simulink model "hdv_hydroelectropowertrain_model"  (R2026a)
settings: Solver=ode1be  StopTime=simulation_length  FixedStep=tsample  MaxStep=tsample
undefined symbols (not defined in the file): alpha, Apump, available_torque, Bpump, btheta_shaft, C1, consumption, Cpump, dp_lim, E0, E1, E2, E3, E_1, Elog, eta_v_m, eta_v_p, ki_dp_comp, ki_te_comp, kp_ctrl_m, kp_dp_comp, kp_te_comp, Kpump, load_blade_enable, Lpump, M, magnitude, Ncell, Npump, omega_e_rpm_ref, omega_l_max_rpm, q1Kalman, q2Kalman, q3Kalman, Qhr, R0, R1, R_tg, rKalman, rpm_base, rpm_consumption, simulation_length, tau_load, tau_load_max, Tc, torque_base, torque_consumption, torque_friction_base, tsample, v_track1_ref, v_track2_ref, valve_mmorifice_max, xv_m_max
libraries: fl_lib x383, nesl_utility x162, linear_swashplate_ctrl_lib x8, flexshaft_lib x5, bichamber_piston_lib x5, variable_displacement_motor_lib x4, variable_displacement_pump_lib x4, fixed_displacement_pump_lib x4, relief_valve_lib x4, inverse_shuttle_valve_lib x4, hydrostatic_threeway_valve_bichamber_piston_lib x4, hydrostatic_fourway_valve_bichamber_piston_lib x4
(part 4 of 8)

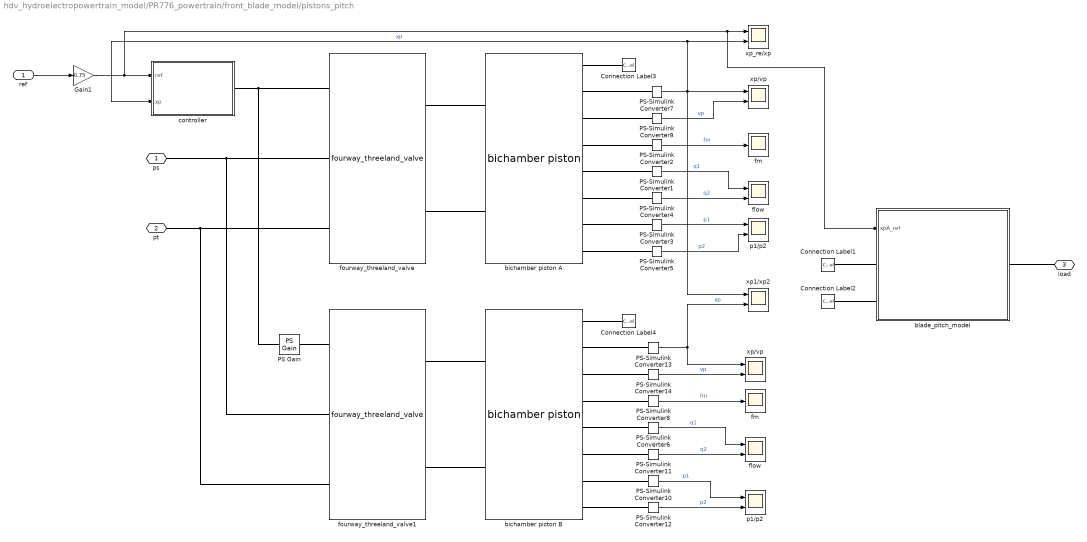
== system hdv_hydroelectropowertrain_model/PR776_powertrain/front_blade_model/pistons_pitch ==
  ref : Inport
  Connection Label1 : ConnectionLabel  Label=A
  Connection Label2 : ConnectionLabel  Label=B
  Connection Label3 : ConnectionLabel  Label=A
  Connection Label4 : ConnectionLabel  Label=B
  Gain1 : Gain  Gain=0.75
  PS Gain : fl_lib/Physical Signals/Functions/PS Gain  gain=-1
  PS-Simulink Converter{1..14} (14 alike) : nesl_utility/PS-Simulink Converter  PhysicalDomain=network_engine_domain  SubClassName=ps_output  LeftPortType=input  RightPortType=output  PseudoPeriodic=off  Frequencies=[]  VectorFormat=1-D array  Unit=inherit  AffineConversion=off
  bichamber piston A : bichamber_piston_lib/bichamber piston  A1=8e-3 m^2  A2=8e-3 m^2  Lp=1.1 m  mp=35 kg  kp=0 N/m  bp=1e3 N/(m/s)  V0=12 l  q1_specify=off  q1_priority=None  q1=0 m^3/s  q1_nominal_specify=off  q1_nominal_value=1  q1_nominal_unit=m^3/s  q2_specify=off  q2_priority=None  q2=0 m^3/s  q2_nominal_specify=off  q2_nominal_value=1  q2_nominal_unit=m^3/s  p1_specify=off  p1_priority=High  p1=0 bar  p1_nominal_specify=off  p1_nominal_value=1  p1_nominal_unit=bar  p2_specify=off  p2_priority=High  p2=0 bar  p2_nominal_specify=off  p2_nominal_value=1  p2_nominal_unit=bar  fp_specify=off  fp_priority=None  fp=0 N  fp_nominal_specify=off  fp_nominal_value=1  fp_nominal_unit=N  vp_specify=off  vp_priority=None  vp=0 m/s  vp_nominal_specify=off  vp_nominal_value=1  vp_nominal_unit=m/s  xp_specify=off  xp_priority=High  xp=0 m  xp_nominal_specify=off  xp_nominal_value=1  xp_nominal_unit=m
  bichamber piston B : bichamber_piston_lib/bichamber piston  A1=8e-3 m^2  A2=8e-3 m^2  Lp=1.1 m  mp=35 kg  kp=0 N/m  bp=1e3 N/(m/s)  V0=12 l  q1_specify=off  q1_priority=None  q1=0 m^3/s  q1_nominal_specify=off  q1_nominal_value=1  q1_nominal_unit=m^3/s  q2_specify=off  q2_priority=None  q2=0 m^3/s  q2_nominal_specify=off  q2_nominal_value=1  q2_nominal_unit=m^3/s  p1_specify=off  p1_priority=High  p1=0 bar  p1_nominal_specify=off  p1_nominal_value=1  p1_nominal_unit=bar  p2_specify=off  p2_priority=High  p2=0 bar  p2_nominal_specify=off  p2_nominal_value=1  p2_nominal_unit=bar  fp_specify=off  fp_priority=None  fp=0 N  fp_nominal_specify=off  fp_nominal_value=1  fp_nominal_unit=N  vp_specify=off  vp_priority=None  vp=0 m/s  vp_nominal_specify=off  vp_nominal_value=1  vp_nominal_unit=m/s  xp_specify=off  xp_priority=High  xp=0 m  xp_nominal_specify=off  xp_nominal_value=1  xp_nominal_unit=m
  blade_pitch_model : Subsystem
  controller : Subsystem
  flow : Scope  NumInputPorts=2
      settings: ActiveDisplayYMinimum=-390.093  ActiveDisplayYMaximum=390.1347
  "flow " : Scope  NumInputPorts=2
      settings: ActiveDisplayYMinimum=-390.093  ActiveDisplayYMaximum=390.1347
  fm : Scope
      settings: ActiveDisplayYMinimum=-672.90251  ActiveDisplayYMaximum=953.14819  DataLoggingVariableName=ScopeData2
  "fm " : Scope
      settings: ActiveDisplayYMinimum=-12251.54126  ActiveDisplayYMaximum=12272.93523  DataLoggingVariableName=ScopeData2
  fourway_threeland_valve : fourway_threeland_valve_lib/fourway_threeland_valve  xv_max=valve_mmorifice_max mm  q1_specify=off  q1_priority=None  q1=0 m^3/s  q1_nominal_specify=off  q1_nominal_unit=m^3/s  q1_nominal_value=1  q2_specify=off  q2_priority=None  q2=0 m^3/s  q2_nominal_specify=off  q2_nominal_unit=m^3/s  q2_nominal_value=1  qin_specify=off  qin_priority=None  qin=0 m^3/s  qin_nominal_specify=off  qin_nominal_unit=m^3/s  qin_nominal_value=1  qout_specify=off  qout_priority=None  qout=0 m^3/s  qout_nominal_specify=off  qout_nominal_unit=m^3/s  qout_nominal_value=1  p1_specify=off  p1_priority=None  p1=0 bar  p1_nominal_specify=off  p1_nominal_unit=bar  p1_nominal_value=1  p2_specify=off  p2_priority=None  p2=0 bar  p2_nominal_specify=off  p2_nominal_unit=bar  p2_nominal_value=1  ps_specify=off  ps_priority=None  ps=0 bar  ps_nominal_specify=off  ps_nominal_unit=bar  ps_nominal_value=1  pt_specify=off  pt_priority=None  pt=0 bar  pt_nominal_specify=off  pt_nominal_unit=bar  pt_nominal_value=1
  fourway_threeland_valve1 : fourway_threeland_valve_lib/fourway_threeland_valve  xv_max=valve_mmorifice_max mm  q1_specify=off  q1_priority=None  q1=0 m^3/s  q1_nominal_specify=off  q1_nominal_unit=m^3/s  q1_nominal_value=1  q2_specify=off  q2_priority=None  q2=0 m^3/s  q2_nominal_specify=off  q2_nominal_unit=m^3/s  q2_nominal_value=1  qin_specify=off  qin_priority=None  qin=0 m^3/s  qin_nominal_specify=off  qin_nominal_unit=m^3/s  qin_nominal_value=1  qout_specify=off  qout_priority=None  qout=0 m^3/s  qout_nominal_specify=off  qout_nominal_unit=m^3/s  qout_nominal_value=1  p1_specify=off  p1_priority=None  p1=0 bar  p1_nominal_specify=off  p1_nominal_unit=bar  p1_nominal_value=1  p2_specify=off  p2_priority=None  p2=0 bar  p2_nominal_specify=off  p2_nominal_unit=bar  p2_nominal_value=1  ps_specify=off  ps_priority=None  ps=0 bar  ps_nominal_specify=off  ps_nominal_unit=bar  ps_nominal_value=1  pt_specify=off  pt_priority=None  pt=0 bar  pt_nominal_specify=off  pt_nominal_unit=bar  pt_nominal_value=1
  p1/p2 : Scope  NumInputPorts=2
      settings: ActiveDisplayYMinimum=-46.741  ActiveDisplayYMaximum=145.78787  DataLoggingVariableName=ScopeData4
  "p1/p2 " : Scope  NumInputPorts=2
      settings: ActiveDisplayYMinimum=-538.19348  ActiveDisplayYMaximum=761.65919  DataLoggingVariableName=ScopeData3
  xp/vp : Scope  NumInputPorts=2
      settings: ActiveDisplayYMinimum=-0.08067  ActiveDisplayYMaximum=1.22604
  "xp/vp " : Scope  NumInputPorts=2
      settings: ActiveDisplayYMinimum=0.8942  ActiveDisplayYMaximum=1.45218  DataLoggingVariableName=ScopeData4
  xp1/xp2 : Scope  NumInputPorts=2
      settings: ActiveDisplayYMinimum=-0.46875  ActiveDisplayYMaximum=0.46875  DataLoggingVariableName=ScopeData6
  xp_re/xp : Scope  NumInputPorts=2
      settings: ActiveDisplayYMinimum=-0.125  ActiveDisplayYMaximum=1.125  DataLoggingVariableName=ScopeData7
  ps : PMIOPort  Side=Left
  pt : PMIOPort  Port=2  Side=Left
  load : PMIOPort  Port=3  Side=Right
  wires:
  PS-Simulink Converter10/1 -> "p1/p2 "/1  "p1"
  PS-Simulink Converter13/1 -> xp1/xp2/2, "xp/vp "/1  "xp"
  PS-Simulink Converter11/1 -> "flow "/2  "q2"
  PS-Simulink Converter14/1 -> "xp/vp "/2  "vp"
  PS-Simulink Converter12/1 -> "p1/p2 "/2  "p2"
  PS-Simulink Converter6/1 -> "flow "/1  "q1"
  PS-Simulink Converter8/1 -> "fm "/1  "fm"
  PS-Simulink Converter2/1 -> fm/1  "fm"
  PS-Simulink Converter1/1 -> flow/1  "q1"
  PS-Simulink Converter5/1 -> p1/p2/2  "p2"
  PS-Simulink Converter9/1 -> xp/vp/2  "vp"
  PS-Simulink Converter4/1 -> flow/2  "q2"
  PS-Simulink Converter7/1 -> xp1/xp2/1, xp/vp/1, controller/2(xp), xp_re/xp/2  "xp"
  PS-Simulink Converter3/1 -> p1/p2/1  "p1"
  ref/1 -> Gain1/1
  Gain1/1 -> controller/1(ref), blade_pitch_model/1(xpA_ref), xp_re/xp/1
  connections:
  bichamber piston B/RConn6 -- PS-Simulink Converter11/LConn1
  bichamber piston B/RConn3 -- PS-Simulink Converter14/LConn1
  bichamber piston B/RConn2 -- PS-Simulink Converter13/LConn1
  bichamber piston B/RConn4 -- PS-Simulink Converter8/LConn1
  bichamber piston B/RConn8 -- PS-Simulink Converter12/LConn1
  bichamber piston B/RConn5 -- PS-Simulink Converter6/LConn1
  bichamber piston B/RConn7 -- PS-Simulink Converter10/LConn1
  fourway_threeland_valve/LConn1 -- PS Gain/LConn1 -- controller/RConn1
  pt/RConn1 -- fourway_threeland_valve/LConn3 -- fourway_threeland_valve1/LConn3
  ps/RConn1 -- fourway_threeland_valve/LConn2 -- fourway_threeland_valve1/LConn2
  bichamber piston A/RConn8 -- PS-Simulink Converter5/LConn1
  bichamber piston A/RConn7 -- PS-Simulink Converter3/LConn1
  bichamber piston A/RConn6 -- PS-Simulink Converter4/LConn1
  bichamber piston A/RConn5 -- PS-Simulink Converter1/LConn1
  bichamber piston A/RConn4 -- PS-Simulink Converter2/LConn1
  bichamber piston A/RConn2 -- PS-Simulink Converter7/LConn1
  bichamber piston A/LConn1 -- fourway_threeland_valve/RConn1
  bichamber piston A/LConn2 -- fourway_threeland_valve/RConn2
  PS Gain/RConn1 -- fourway_threeland_valve1/LConn1
  bichamber piston A/RConn3 -- PS-Simulink Converter9/LConn1
  fourway_threeland_valve1/RConn1 -- bichamber piston B/LConn1
  fourway_threeland_valve1/RConn2 -- bichamber piston B/LConn2
  Connection Label3/LConn1 -- bichamber piston A/RConn1
  bichamber piston B/RConn1 -- Connection Label4/LConn1
  Connection Label1/LConn1 -- blade_pitch_model/LConn1
  Connection Label2/LConn1 -- blade_pitch_model/LConn2
  blade_pitch_model/RConn1 -- load/RConn1

== system hdv_hydroelectropowertrain_model/PR776_powertrain/front_blade_model/pitch_load ==
  Simulink-PS Converter1 : nesl_utility/Simulink-PS Converter  PhysicalDomain=network_engine_domain  SubClassName=ps_input  LeftPortType=input  RightPortType=output  PseudoPeriodic=off  Frequencies=[]  NoiseDistribution=none  NoiseParameters=[]  Unit=N  AffineConversion=on  FilteringAndDerivatives=provide  SimscapeFilterOrder=1  InputFilterTimeConstant=0.001  UdotUserProvided=0
  "pitch_load  " : Subsystem
  load : PMIOPort  Side=Right
  wires:
  "pitch_load  "/1(Out1) -> Simulink-PS Converter1/1  "pitch_load"
  connections:
  load/RConn1 -- Simulink-PS Converter1/RConn1

== system hdv_hydroelectropowertrain_model/PR776_powertrain/front_blade_model/tilt_load ==
  Simulink-PS Converter1 : nesl_utility/Simulink-PS Converter  PhysicalDomain=network_engine_domain  SubClassName=ps_input  LeftPortType=input  RightPortType=output  PseudoPeriodic=off  Frequencies=[]  NoiseDistribution=none  NoiseParameters=[]  Unit=N  AffineConversion=on  FilteringAndDerivatives=provide  SimscapeFilterOrder=1  InputFilterTimeConstant=0.001  UdotUserProvided=0
  "tilt_load  " : Subsystem
  load : PMIOPort  Side=Right
  wires:
  "tilt_load  "/1(Out1) -> Simulink-PS Converter1/1  "tilt_load"
  connections:
  load/RConn1 -- Simulink-PS Converter1/RConn1

== system hdv_hydroelectropowertrain_model/PR776_powertrain/front_blade_model/vertical_load ==
  Blade_load : fl_lib/Mechanical/Mechanical Sources/Ideal Force Source
  Constant : Constant  Value=31878
  Mechanical Translational Reference : fl_lib/Mechanical/Translational Elements/Mechanical Translational Reference
  Simulink-PS Converter1 : nesl_utility/Simulink-PS Converter  PhysicalDomain=network_engine_domain  SubClassName=ps_input  LeftPortType=input  RightPortType=output  PseudoPeriodic=off  Frequencies=[]  NoiseDistribution=none  NoiseParameters=[]  Unit=N  AffineConversion=on  FilteringAndDerivatives=provide  SimscapeFilterOrder=1  InputFilterTimeConstant=0.001  UdotUserProvided=0
  To Workspace6 : ToWorkspace  VariableName=sim_load  SampleTime=Tc
      settings: MaxDataPoints=Nc
  load : Scope
      settings: ActiveDisplayYMinimum=-19625  ActiveDisplayYMaximum=176625  DataLoggingVariableName=ScopeData3
  load_disturbance : Subsystem
  vertical_load : PMIOPort  Side=Left
  wires:
  load_disturbance/1(Out1) -> load/1, To Workspace6/1  "load_force"
  Constant/1 -> Simulink-PS Converter1/1
  connections:
  Mechanical Translational Reference/LConn1 -- Blade_load/RConn2
  Simulink-PS Converter1/RConn1 -- Blade_load/RConn1
  vertical_load/RConn1 -- Blade_load/LConn1

== system hdv_hydroelectropowertrain_model/Vehicle Control System/Engine Anti-Stall/Engine Overload Control ==
  x : Inport
  xref : Inport  Port=2
  1/Ti : Gain  Gain=kp  SaturateOnIntegerOverflow=on  OutDataTypeStr=Inherit: Same as input  ParamDataTypeStr=Inherit: Same as input
  Saturation : Saturate  UpperLimit=sat_pos  LowerLimit=sat_neg
  Sum1 : Sum  Inputs=+++  SaturateOnIntegerOverflow=on
  Sum2 : Sum  Inputs=-+  SaturateOnIntegerOverflow=on
  Sum3 : Sum  Inputs=-+  SaturateOnIntegerOverflow=on
  Unit Delay4 : UnitDelay  SampleTime=tsample
  kp : Gain  Gain=ki*ts  SaturateOnIntegerOverflow=on  OutDataTypeStr=Inherit: Same as input  ParamDataTypeStr=Inherit: Same as input
  u : Outport
  wires:
  Saturation/1 -> Sum3/2, u/1
  Unit Delay4/1 -> Sum1/3
  Sum1/1 -> Saturation/1
  x/1 -> Sum2/1
  Sum3/1 -> Unit Delay4/1
  1/Ti/1 -> Sum3/1, Sum1/1
  Sum2/1 -> 1/Ti/1, kp/1
  kp/1 -> Sum1/2
  xref/1 -> Sum2/2

== system hdv_hydroelectropowertrain_model/Vehicle Control System/Over Pressure Compensation/Pressure Compensation Control A ==
  x : Inport
  xref : Inport  Port=2
  1/Ti : Gain  Gain=kp  SaturateOnIntegerOverflow=on  OutDataTypeStr=Inherit: Same as input  ParamDataTypeStr=Inherit: Same as input
  Saturation : Saturate  UpperLimit=sat_pos  LowerLimit=sat_neg
  Sum1 : Sum  Inputs=+++  SaturateOnIntegerOverflow=on
  Sum2 : Sum  Inputs=-+  SaturateOnIntegerOverflow=on
  Sum3 : Sum  Inputs=-+  SaturateOnIntegerOverflow=on
  Unit Delay4 : UnitDelay  SampleTime=tsample
  kp : Gain  Gain=ki*ts  SaturateOnIntegerOverflow=on  OutDataTypeStr=Inherit: Same as input  ParamDataTypeStr=Inherit: Same as input
  u : Outport
  wires:
  xref/1 -> Sum2/2
  kp/1 -> Sum1/2
  1/Ti/1 -> Sum1/1, Sum3/1
  Sum3/1 -> Unit Delay4/1
  x/1 -> Sum2/1
  Sum1/1 -> Saturation/1
  Unit Delay4/1 -> Sum1/3
  Saturation/1 -> u/1, Sum3/2
  Sum2/1 -> 1/Ti/1, kp/1

== system hdv_hydroelectropowertrain_model/Vehicle Control System/Over Pressure Compensation/Pressure Compensation Control B ==
  x : Inport
  xref : Inport  Port=2
  1/Ti : Gain  Gain=kp  SaturateOnIntegerOverflow=on  OutDataTypeStr=Inherit: Same as input  ParamDataTypeStr=Inherit: Same as input
  Saturation : Saturate  UpperLimit=sat_pos  LowerLimit=sat_neg
  Sum1 : Sum  Inputs=+++  SaturateOnIntegerOverflow=on
  Sum2 : Sum  Inputs=-+  SaturateOnIntegerOverflow=on
  Sum3 : Sum  Inputs=-+  SaturateOnIntegerOverflow=on
  Unit Delay4 : UnitDelay  SampleTime=tsample
  kp : Gain  Gain=ki*ts  SaturateOnIntegerOverflow=on  OutDataTypeStr=Inherit: Same as input  ParamDataTypeStr=Inherit: Same as input
  u : Outport
  wires:
  Saturation/1 -> Sum3/2, u/1
  Unit Delay4/1 -> Sum1/3
  Sum1/1 -> Saturation/1
  x/1 -> Sum2/1
  Sum3/1 -> Unit Delay4/1
  1/Ti/1 -> Sum3/1, Sum1/1
  Sum2/1 -> 1/Ti/1, kp/1
  kp/1 -> Sum1/2
  xref/1 -> Sum2/2

== system hdv_hydroelectropowertrain_model/Vehicle Control System/Over Pressure Compensation/direction1 ==
  In1 : Inport
  Product : Product
  Out1 : Outport
  wires:
  In1/1 -> Product/1
  Product/1 -> Out1/1
  [direction_RT] -> Product/2

== system hdv_hydroelectropowertrain_model/Vehicle Control System/Over Pressure Compensation/direction2 ==
  In1 : Inport
  Product : Product
  Out1 : Outport
  wires:
  Product/1 -> Out1/1
  In1/1 -> Product/1
  [direction_LT] -> Product/2

== system hdv_hydroelectropowertrain_model/Vehicle Control System/lineA_compensations/direction_RT ==
  In1 : Inport
  Product : Product
  ETComp : Outport
  wires:
  Product/1 -> ETComp/1
  In1/1 -> Product/1
  [direction_RT] -> Product/2

== system hdv_hydroelectropowertrain_model/Vehicle Control System/lineB_compensations /direction_LT ==
  In1 : Inport
  Product : Product
  ETComp : Outport
  wires:
  Product/1 -> ETComp/1
  In1/1 -> Product/1
  [direction_LT] -> Product/2

== system hdv_hydroelectropowertrain_model/Vehicle Control System/synch_overspeed_management/Maximum Speed Control ==
  x : Inport
  xref : Inport  Port=2
  1/Ti : Gain  Gain=kp  SaturateOnIntegerOverflow=on  OutDataTypeStr=Inherit: Same as input  ParamDataTypeStr=Inherit: Same as input
  Saturation : Saturate  UpperLimit=sat_pos  LowerLimit=sat_neg
  Sum1 : Sum  Inputs=+++  SaturateOnIntegerOverflow=on
  Sum2 : Sum  Inputs=-+  SaturateOnIntegerOverflow=on
  Sum3 : Sum  Inputs=-+  SaturateOnIntegerOverflow=on
  Unit Delay4 : UnitDelay  SampleTime=ts
  direction_lineA : Subsystem
  kp : Gain  Gain=ki*tsample  SaturateOnIntegerOverflow=on  OutDataTypeStr=Inherit: Same as input  ParamDataTypeStr=Inherit: Same as input
  u : Outport
  wires:
  xref/1 -> Sum2/2
  kp/1 -> Sum1/2
  1/Ti/1 -> Sum1/1, Sum3/1
  Sum3/1 -> Unit Delay4/1
  x/1 -> Sum2/1
  Sum1/1 -> Saturation/1
  Unit Delay4/1 -> Sum1/3
  Saturation/1 -> direction_lineA/1(In1), Sum3/2
  Sum2/1 -> kp/1, 1/Ti/1
  direction_lineA/1(u) -> u/1

== system hdv_hydroelectropowertrain_model/Vehicle Control System/synch_overspeed_management/Steering Reference Control ==
  x : Inport
  xref : Inport  Port=2
  1/Ti : Gain  Gain=kp  SaturateOnIntegerOverflow=on  OutDataTypeStr=Inherit: Same as input  ParamDataTypeStr=Inherit: Same as input
  Saturation : Saturate  UpperLimit=sat_pos  LowerLimit=sat_neg
  Sum1 : Sum  Inputs=+++  SaturateOnIntegerOverflow=on
  Sum2 : Sum  Inputs=-+  SaturateOnIntegerOverflow=on
  Sum3 : Sum  Inputs=-+  SaturateOnIntegerOverflow=on
  Unit Delay4 : UnitDelay  SampleTime=tsample
  kp : Gain  Gain=ki*ts  SaturateOnIntegerOverflow=on  OutDataTypeStr=Inherit: Same as input  ParamDataTypeStr=Inherit: Same as input
  u : Outport
  wires:
  Saturation/1 -> Sum3/2, u/1
  Unit Delay4/1 -> Sum1/3
  Sum1/1 -> Saturation/1
  x/1 -> Sum2/1
  Sum3/1 -> Unit Delay4/1
  1/Ti/1 -> Sum3/1, Sum1/1
  Sum2/1 -> 1/Ti/1, kp/1
  kp/1 -> Sum1/2
  xref/1 -> Sum2/2

== system hdv_hydroelectropowertrain_model/PR776_powertrain/Hydrostatic_powertrain/driveine_LD1/pressure_charge_system_LD ==
  Hydraulic Flow Rate Sensor : fl_lib/Hydraulic/Hydraulic Sensors/Hydraulic Flow Rate Sensor
  Hydraulic Flow Rate Sensor1 : fl_lib/Hydraulic/Hydraulic Sensors/Hydraulic Flow Rate Sensor
  Hydraulic Pressure Sensor{1..4} (4 alike) : fl_lib/Hydraulic/Hydraulic Sensors/Hydraulic Pressure Sensor
  Hydraulic Reference1 : fl_lib/Hydraulic/Hydraulic Elements/Hydraulic Reference
  Hydraulic Reference2 : fl_lib/Hydraulic/Hydraulic Elements/Hydraulic Reference
  Hydraulic Reference3 : fl_lib/Hydraulic/Hydraulic Elements/Hydraulic Reference
  Mux : Mux  Inputs=2
  PS-Simulink Converter : nesl_utility/PS-Simulink Converter  PhysicalDomain=network_engine_domain  SubClassName=ps_output  LeftPortType=input  RightPortType=output  PseudoPeriodic=off  Frequencies=[]  VectorFormat=1-D array  Unit=l/min  AffineConversion=on
  PS-Simulink Converter{1..3,5} (4 alike) : nesl_utility/PS-Simulink Converter  PhysicalDomain=network_engine_domain  SubClassName=ps_output  LeftPortType=input  RightPortType=output  PseudoPeriodic=off  Frequencies=[]  VectorFormat=1-D array  Unit=bar  AffineConversion=on
  PS-Simulink Converter4 : nesl_utility/PS-Simulink Converter  PhysicalDomain=network_engine_domain  SubClassName=ps_output  LeftPortType=input  RightPortType=output  PseudoPeriodic=off  Frequencies=[]  VectorFormat=1-D array  Unit=l/min  AffineConversion=on
  Scope1 : Scope  NumInputPorts=2
      settings: SampleTime=tsample  ActiveDisplayYMinimum=-171.1725  ActiveDisplayYMaximum=527.07344  DataLoggingVariableName=ScopeData2
  Scope2 : Scope  NumInputPorts=2
      settings: SampleTime=tsample  ActiveDisplayYMinimum=-2.39042  ActiveDisplayYMaximum=21.51378  DataLoggingVariableName=ScopeData2
  Scope3 : Scope  NumInputPorts=2
      settings: SampleTime=tsample  ActiveDisplayYMinimum=-2.35304  ActiveDisplayYMaximum=21.17734
  Subsystem : Subsystem
  hydro_check_valve1 : Subsystem
      settings: PortSchema="{\"entries\":[{\"content\":{\"sides\":[{\"content\":{\"connectorIds\":[]},\"type\":\"ConnectorPlacement.EquallySpacedRectSide\",\"uuid\":\"a69fbb91-2279-4dfd-af6f-16497d5f1538\"},{\"content\":{\"connectorIds\":[],\"side\":\"RIGHT\"},\"type\":\"ConnectorPlacement.EquallySpacedRectSide\",\"uuid\":\"52e95d44-b7af-4ccc-8556-a2abd2e724e0\"},{\"content\":{\"connectorIds\":[\"LConn1\"],\"side\":\"TOP\"},\"type\":\"ConnectorPlacement.EquallySpacedRectSide\",\"uuid\":\"2d8c071e-4cd0-4b83-8d45-c175cb858754\"},{\"content\":{\"connectorIds\":[\"RConn1\"],\"side\":\"BOTTOM\"},\"type\":\"ConnectorPlacement.EquallySpacedRectSide\",\"uuid\":\"1baec9dc-757c-4f21-904a-6fc08de72ce1\"}]},\"type\":\"ConnectorPlacement.EquallySpacedConnector\",\"uuid\":\"76990e53-6cb0-4bfe-8c9e-427c41b785f2\"}],\"packageUris\":[\"http://schema.mathworks.com/mf0/Connector/19700101\"],\"version\":\"1.0\"}"
  hydro_check_valve2 : Subsystem
      settings: PortSchema="{\"entries\":[{\"content\":{\"sides\":[{\"content\":{\"connectorIds\":[]},\"type\":\"ConnectorPlacement.EquallySpacedRectSide\",\"uuid\":\"a69fbb91-2279-4dfd-af6f-16497d5f1538\"},{\"content\":{\"connectorIds\":[],\"side\":\"RIGHT\"},\"type\":\"ConnectorPlacement.EquallySpacedRectSide\",\"uuid\":\"52e95d44-b7af-4ccc-8556-a2abd2e724e0\"},{\"content\":{\"connectorIds\":[\"LConn1\"],\"side\":\"TOP\"},\"type\":\"ConnectorPlacement.EquallySpacedRectSide\",\"uuid\":\"2d8c071e-4cd0-4b83-8d45-c175cb858754\"},{\"content\":{\"connectorIds\":[\"RConn1\"],\"side\":\"BOTTOM\"},\"type\":\"ConnectorPlacement.EquallySpacedRectSide\",\"uuid\":\"1baec9dc-757c-4f21-904a-6fc08de72ce1\"}]},\"type\":\"ConnectorPlacement.EquallySpacedConnector\",\"uuid\":\"76990e53-6cb0-4bfe-8c9e-427c41b785f2\"}],\"packageUris\":[\"http://schema.mathworks.com/mf0/Connector/19700101\"],\"version\":\"1.0\"}"
  inverse shuttle valve : inverse_shuttle_valve_lib/inverse shuttle valve  pnom=32 bar  dp_crack=0 bar  dp_reg=0 bar  x_rv_max=2 mm  a0=(2*pi*10)^2 1/s^2  a1=2*2*pi*10 1/s  leak=5e-12 m^3/s/Pa  qA_specify=off  qA_priority=None  qA=0 m^3/s  qA_nominal_specify=off  qA_nominal_unit=m^3/s  qA_nominal_value=1  qB_specify=off  qB_priority=None  qB=0 m^3/s  qB_nominal_specify=off  qB_nominal_unit=m^3/s  qB_nominal_value=1  qP_specify=off  qP_priority=None  qP=0 m^3/s  qP_nominal_specify=off  qP_nominal_unit=m^3/s  qP_nominal_value=1  dp_specify=off  dp_priority=None  dp=0 Pa  dp_nominal_specify=off  dp_nominal_unit=Pa  dp_nominal_value=1  dpAP_specify=off  dpAP_priority=None  dpAP=0 Pa  dpAP_nominal_specify=off  dpAP_nominal_unit=Pa  dpAP_nominal_value=1  dpBP_specify=off  dpBP_priority=None  dpBP=0 Pa  dpBP_nominal_specify=off  dpBP_nominal_unit=Pa  dpBP_nominal_value=1  x_rv_AP_specify=off  x_rv_AP_priority=None  x_rv_AP=0 m  x_rv_AP_nominal_specify=off  x_rv_AP_nominal_unit=m  x_rv_AP_nominal_value=1  x_rv_BP_specify=off  x_rv_BP_priority=None  x_rv_BP=0 m  x_rv_BP_nominal_specify=off  x_rv_BP_nominal_unit=m  x_rv_BP_nominal_value=1  x_rv_AP_flt_specify=off  x_rv_AP_flt_priority=None  x_rv_AP_flt=0 m  x_rv_AP_flt_nominal_specify=off  x_rv_AP_flt_nominal_unit=m  x_rv_AP_flt_nominal_value=1  x_rv_BP_flt_specify=off  x_rv_BP_flt_priority=None  x_rv_BP_flt=0 m  x_rv_BP_flt_nominal_specify=off  x_rv_BP_flt_nominal_unit=m  x_rv_BP_flt_nominal_value=1
  A : PMIOPort  Side=Left
  B : PMIOPort  Port=2  Side=Right
  D : PMIOPort  Port=3  Side=Right
  wires:
  PS-Simulink Converter5/1 -> Scope3/2  "dp"
  PS-Simulink Converter4/1 -> Scope3/1  "qT_ishuttle"
  PS-Simulink Converter3/1 -> Scope2/2  "pCharge"
  PS-Simulink Converter/1 -> Scope1/2, Scope2/1  "qcharge"
  Mux/1 -> Scope1/1
  PS-Simulink Converter1/1 -> Mux/1  "pB"
  PS-Simulink Converter2/1 -> Mux/2  "pA"
  connections:
  PS-Simulink Converter5/LConn1 -- Hydraulic Pressure Sensor4/RConn2
  Hydraulic Flow Rate Sensor1/RConn1 -- PS-Simulink Converter4/LConn1
  Hydraulic Flow Rate Sensor1/RConn2 -- Hydraulic Reference3/LConn1
  Hydraulic Reference2/LConn1 -- Hydraulic Pressure Sensor3/RConn1
  Hydraulic Pressure Sensor3/RConn2 -- PS-Simulink Converter3/LConn1
  Subsystem/LConn1 -- D/RConn1
  Hydraulic Flow Rate Sensor/LConn1 -- Subsystem/RConn1 -- Hydraulic Pressure Sensor3/LConn1
  Hydraulic Flow Rate Sensor/RConn1 -- PS-Simulink Converter/LConn1
  Hydraulic Pressure Sensor2/RConn2 -- PS-Simulink Converter2/LConn1
  Hydraulic Pressure Sensor1/RConn2 -- PS-Simulink Converter1/LConn1
  Hydraulic Pressure Sensor1/RConn1 -- Hydraulic Reference1/LConn1 -- Hydraulic Pressure Sensor2/RConn1
  Hydraulic Pressure Sensor4/RConn1 -- Hydraulic Pressure Sensor1/LConn1 -- B/RConn1 -- inverse shuttle valve/LConn2 -- hydro_check_valve2/RConn1
  Hydraulic Pressure Sensor4/LConn1 -- Hydraulic Pressure Sensor2/LConn1 -- A/RConn1 -- inverse shuttle valve/LConn1 -- hydro_check_valve1/RConn1
  hydro_check_valve1/LConn1 -- Hydraulic Flow Rate Sensor/RConn2 -- hydro_check_valve2/LConn1
  inverse shuttle valve/RConn1 -- Hydraulic Flow Rate Sensor1/LConn1

== system hdv_hydroelectropowertrain_model/PR776_powertrain/Hydrostatic_powertrain/driveine_LD1/vd_ctrl_motor_LD ==
  vd_ref : Inport
  Linear swashplate ctrl2 : linear_swashplate_ctrl_lib/Linear swashplate ctrl  Commented=on  a12=1 1/s  b2=1 1/m/s  k1=100 m  k2=20.5 m  N=5 m  kv=20  xv_specify=off  xv_priority=None  xv=0 m  xv_nominal_specify=off  xv_nominal_unit=m  xv_nominal_value=1  D1_specify=off  D1_priority=None  D1=0  D1_nominal_specify=off  D1_nominal_unit=1  D1_nominal_value=1  D2_specify=off  D2_priority=None  D2=0  D2_nominal_specify=off  D2_nominal_unit=1  D2_nominal_value=1
  PS-Simulink Converter : nesl_utility/PS-Simulink Converter  PhysicalDomain=network_engine_domain  SubClassName=ps_output  LeftPortType=input  RightPortType=output  PseudoPeriodic=off  Frequencies=[]  VectorFormat=1-D array  Unit=inherit  AffineConversion=off
  Scope : Scope  NumInputPorts=2
      settings: ActiveDisplayYMinimum=0.29414  ActiveDisplayYMaximum=1.07846  DataLoggingVariableName=ScopeData3
  Simulink-PS Converter3 : nesl_utility/Simulink-PS Converter  Commented=on  PhysicalDomain=network_engine_domain  SubClassName=ps_input  LeftPortType=input  RightPortType=output  PseudoPeriodic=off  Frequencies=[]  NoiseDistribution=none  NoiseParameters=[]  Unit=1  AffineConversion=off  FilteringAndDerivatives=provide  SimscapeFilterOrder=1  InputFilterTimeConstant=0.001  UdotUserProvided=0
  hose3 : Subsystem
  servo motor LD : Subsystem
  vd : PMIOPort  Side=Right
  pS : PMIOPort  Port=2  Side=Left
  pT : PMIOPort  Port=3  Side=Left
  wires:
  PS-Simulink Converter/1 -> Scope/2
  vd_ref/1 -> servo motor LD/1(displacement reference pu), Scope/1, Simulink-PS Converter3/1
  connections:
  Simulink-PS Converter3/RConn1 -- Linear swashplate ctrl2/LConn1
  pS/RConn1 -- hose3/LConn1
  pT/RConn1 -- hose3/LConn2
  hose3/RConn1 -- servo motor LD/LConn1
  hose3/RConn2 -- servo motor LD/LConn2
  servo motor LD/RConn1 -- PS-Simulink Converter/LConn1 -- vd/RConn1

== system hdv_hydroelectropowertrain_model/PR776_powertrain/Hydrostatic_powertrain/driveine_LD1/vd_ctrl_pump_LD ==
  vd_ref : Inport
  Linear swashplate ctrl2 : linear_swashplate_ctrl_lib/Linear swashplate ctrl  Commented=on  a12=1 1/s  b2=1 1/m/s  k1=100 m  k2=20.5 m  N=5 m  kv=20  xv_specify=off  xv_priority=None  xv=0 m  xv_nominal_specify=off  xv_nominal_unit=m  xv_nominal_value=1  D1_specify=off  D1_priority=None  D1=0  D1_nominal_specify=off  D1_nominal_unit=1  D1_nominal_value=1  D2_specify=off  D2_priority=None  D2=0  D2_nominal_specify=off  D2_nominal_unit=1  D2_nominal_value=1
  Simulink-PS Converter3 : nesl_utility/Simulink-PS Converter  Commented=on  PhysicalDomain=network_engine_domain  SubClassName=ps_input  LeftPortType=input  RightPortType=output  PseudoPeriodic=off  Frequencies=[]  NoiseDistribution=none  NoiseParameters=[]  Unit=1  AffineConversion=off  FilteringAndDerivatives=provide  SimscapeFilterOrder=1  InputFilterTimeConstant=0.001  UdotUserProvided=0
  hose3 : Subsystem
  servo pump RD : Subsystem
  vd : PMIOPort  Side=Right
  pS : PMIOPort  Port=2  Side=Left
  pT : PMIOPort  Port=3  Side=Left
  wires:
  vd_ref/1 -> Simulink-PS Converter3/1, servo pump RD/1(displacement reference pu)
  connections:
  pT/RConn1 -- hose3/LConn2
  pS/RConn1 -- hose3/LConn1
  servo pump RD/LConn1 -- hose3/RConn1
  servo pump RD/LConn2 -- hose3/RConn2
  Simulink-PS Converter3/RConn1 -- Linear swashplate ctrl2/LConn1
  servo pump RD/RConn1 -- vd/RConn1

== system hdv_hydroelectropowertrain_model/PR776_powertrain/Hydrostatic_powertrain/driveine_LD2/pressure_charge_system_LD ==
  Hydraulic Flow Rate Sensor : fl_lib/Hydraulic/Hydraulic Sensors/Hydraulic Flow Rate Sensor
  Hydraulic Flow Rate Sensor1 : fl_lib/Hydraulic/Hydraulic Sensors/Hydraulic Flow Rate Sensor
  Hydraulic Pressure Sensor{1..4} (4 alike) : fl_lib/Hydraulic/Hydraulic Sensors/Hydraulic Pressure Sensor
  Hydraulic Reference1 : fl_lib/Hydraulic/Hydraulic Elements/Hydraulic Reference
  Hydraulic Reference2 : fl_lib/Hydraulic/Hydraulic Elements/Hydraulic Reference
  Hydraulic Reference3 : fl_lib/Hydraulic/Hydraulic Elements/Hydraulic Reference
  Mux : Mux  Inputs=2
  PS-Simulink Converter : nesl_utility/PS-Simulink Converter  PhysicalDomain=network_engine_domain  SubClassName=ps_output  LeftPortType=input  RightPortType=output  PseudoPeriodic=off  Frequencies=[]  VectorFormat=1-D array  Unit=l/min  AffineConversion=on
  PS-Simulink Converter{1..3,5} (4 alike) : nesl_utility/PS-Simulink Converter  PhysicalDomain=network_engine_domain  SubClassName=ps_output  LeftPortType=input  RightPortType=output  PseudoPeriodic=off  Frequencies=[]  VectorFormat=1-D array  Unit=bar  AffineConversion=on
  PS-Simulink Converter4 : nesl_utility/PS-Simulink Converter  PhysicalDomain=network_engine_domain  SubClassName=ps_output  LeftPortType=input  RightPortType=output  PseudoPeriodic=off  Frequencies=[]  VectorFormat=1-D array  Unit=l/min  AffineConversion=on
  Scope1 : Scope  NumInputPorts=2
      settings: SampleTime=tsample  ActiveDisplayYMinimum=-171.1725  ActiveDisplayYMaximum=527.07344  DataLoggingVariableName=ScopeData2
  Scope2 : Scope  NumInputPorts=2
      settings: SampleTime=tsample  ActiveDisplayYMinimum=-2.39042  ActiveDisplayYMaximum=21.51378  DataLoggingVariableName=ScopeData2
  Scope3 : Scope  NumInputPorts=2
      settings: SampleTime=tsample  ActiveDisplayYMinimum=-2.35304  ActiveDisplayYMaximum=21.17734
  Subsystem : Subsystem
  hydro_check_valve1 : Subsystem
      settings: PortSchema="{\"entries\":[{\"content\":{\"sides\":[{\"content\":{\"connectorIds\":[]},\"type\":\"ConnectorPlacement.EquallySpacedRectSide\",\"uuid\":\"a69fbb91-2279-4dfd-af6f-16497d5f1538\"},{\"content\":{\"connectorIds\":[],\"side\":\"RIGHT\"},\"type\":\"ConnectorPlacement.EquallySpacedRectSide\",\"uuid\":\"52e95d44-b7af-4ccc-8556-a2abd2e724e0\"},{\"content\":{\"connectorIds\":[\"LConn1\"],\"side\":\"TOP\"},\"type\":\"ConnectorPlacement.EquallySpacedRectSide\",\"uuid\":\"2d8c071e-4cd0-4b83-8d45-c175cb858754\"},{\"content\":{\"connectorIds\":[\"RConn1\"],\"side\":\"BOTTOM\"},\"type\":\"ConnectorPlacement.EquallySpacedRectSide\",\"uuid\":\"1baec9dc-757c-4f21-904a-6fc08de72ce1\"}]},\"type\":\"ConnectorPlacement.EquallySpacedConnector\",\"uuid\":\"76990e53-6cb0-4bfe-8c9e-427c41b785f2\"}],\"packageUris\":[\"http://schema.mathworks.com/mf0/Connector/19700101\"],\"version\":\"1.0\"}"
  hydro_check_valve2 : Subsystem
      settings: PortSchema="{\"entries\":[{\"content\":{\"sides\":[{\"content\":{\"connectorIds\":[]},\"type\":\"ConnectorPlacement.EquallySpacedRectSide\",\"uuid\":\"a69fbb91-2279-4dfd-af6f-16497d5f1538\"},{\"content\":{\"connectorIds\":[],\"side\":\"RIGHT\"},\"type\":\"ConnectorPlacement.EquallySpacedRectSide\",\"uuid\":\"52e95d44-b7af-4ccc-8556-a2abd2e724e0\"},{\"content\":{\"connectorIds\":[\"LConn1\"],\"side\":\"TOP\"},\"type\":\"ConnectorPlacement.EquallySpacedRectSide\",\"uuid\":\"2d8c071e-4cd0-4b83-8d45-c175cb858754\"},{\"content\":{\"connectorIds\":[\"RConn1\"],\"side\":\"BOTTOM\"},\"type\":\"ConnectorPlacement.EquallySpacedRectSide\",\"uuid\":\"1baec9dc-757c-4f21-904a-6fc08de72ce1\"}]},\"type\":\"ConnectorPlacement.EquallySpacedConnector\",\"uuid\":\"76990e53-6cb0-4bfe-8c9e-427c41b785f2\"}],\"packageUris\":[\"http://schema.mathworks.com/mf0/Connector/19700101\"],\"version\":\"1.0\"}"
  inverse shuttle valve : inverse_shuttle_valve_lib/inverse shuttle valve  pnom=32 bar  dp_crack=0 bar  dp_reg=0 bar  x_rv_max=2 mm  a0=(2*pi*10)^2 1/s^2  a1=2*2*pi*10 1/s  leak=5e-12 m^3/s/Pa  qA_specify=off  qA_priority=None  qA=0 m^3/s  qA_nominal_specify=off  qA_nominal_unit=m^3/s  qA_nominal_value=1  qB_specify=off  qB_priority=None  qB=0 m^3/s  qB_nominal_specify=off  qB_nominal_unit=m^3/s  qB_nominal_value=1  qP_specify=off  qP_priority=None  qP=0 m^3/s  qP_nominal_specify=off  qP_nominal_unit=m^3/s  qP_nominal_value=1  dp_specify=off  dp_priority=None  dp=0 Pa  dp_nominal_specify=off  dp_nominal_unit=Pa  dp_nominal_value=1  dpAP_specify=off  dpAP_priority=None  dpAP=0 Pa  dpAP_nominal_specify=off  dpAP_nominal_unit=Pa  dpAP_nominal_value=1  dpBP_specify=off  dpBP_priority=None  dpBP=0 Pa  dpBP_nominal_specify=off  dpBP_nominal_unit=Pa  dpBP_nominal_value=1  x_rv_AP_specify=off  x_rv_AP_priority=None  x_rv_AP=0 m  x_rv_AP_nominal_specify=off  x_rv_AP_nominal_unit=m  x_rv_AP_nominal_value=1  x_rv_BP_specify=off  x_rv_BP_priority=None  x_rv_BP=0 m  x_rv_BP_nominal_specify=off  x_rv_BP_nominal_unit=m  x_rv_BP_nominal_value=1  x_rv_AP_flt_specify=off  x_rv_AP_flt_priority=None  x_rv_AP_flt=0 m  x_rv_AP_flt_nominal_specify=off  x_rv_AP_flt_nominal_unit=m  x_rv_AP_flt_nominal_value=1  x_rv_BP_flt_specify=off  x_rv_BP_flt_priority=None  x_rv_BP_flt=0 m  x_rv_BP_flt_nominal_specify=off  x_rv_BP_flt_nominal_unit=m  x_rv_BP_flt_nominal_value=1
  A : PMIOPort  Side=Left
  B : PMIOPort  Port=2  Side=Right
  D : PMIOPort  Port=3  Side=Right
  wires:
  PS-Simulink Converter2/1 -> Mux/2  "pA"
  PS-Simulink Converter1/1 -> Mux/1  "pB"
  Mux/1 -> Scope1/1
  PS-Simulink Converter/1 -> Scope2/1, Scope1/2  "qcharge"
  PS-Simulink Converter3/1 -> Scope2/2  "pCharge"
  PS-Simulink Converter4/1 -> Scope3/1  "qT_ishuttle"
  PS-Simulink Converter5/1 -> Scope3/2  "dp"
  connections:
  inverse shuttle valve/RConn1 -- Hydraulic Flow Rate Sensor1/LConn1
  hydro_check_valve2/LConn1 -- Hydraulic Flow Rate Sensor/RConn2 -- hydro_check_valve1/LConn1
  hydro_check_valve1/RConn1 -- inverse shuttle valve/LConn1 -- A/RConn1 -- Hydraulic Pressure Sensor2/LConn1 -- Hydraulic Pressure Sensor4/LConn1
  hydro_check_valve2/RConn1 -- inverse shuttle valve/LConn2 -- B/RConn1 -- Hydraulic Pressure Sensor1/LConn1 -- Hydraulic Pressure Sensor4/RConn1
  Hydraulic Pressure Sensor2/RConn1 -- Hydraulic Reference1/LConn1 -- Hydraulic Pressure Sensor1/RConn1
  Hydraulic Pressure Sensor1/RConn2 -- PS-Simulink Converter1/LConn1
  Hydraulic Pressure Sensor2/RConn2 -- PS-Simulink Converter2/LConn1
  Hydraulic Flow Rate Sensor/RConn1 -- PS-Simulink Converter/LConn1
  Hydraulic Pressure Sensor3/LConn1 -- Subsystem/RConn1 -- Hydraulic Flow Rate Sensor/LConn1
  Subsystem/LConn1 -- D/RConn1
  Hydraulic Pressure Sensor3/RConn2 -- PS-Simulink Converter3/LConn1
  Hydraulic Reference2/LConn1 -- Hydraulic Pressure Sensor3/RConn1
  Hydraulic Flow Rate Sensor1/RConn2 -- Hydraulic Reference3/LConn1
  Hydraulic Flow Rate Sensor1/RConn1 -- PS-Simulink Converter4/LConn1
  PS-Simulink Converter5/LConn1 -- Hydraulic Pressure Sensor4/RConn2

== system hdv_hydroelectropowertrain_model/PR776_powertrain/Hydrostatic_powertrain/driveine_LD2/vd_ctrl_motor_LD ==
  vd_ref : Inport
  Linear swashplate ctrl2 : linear_swashplate_ctrl_lib/Linear swashplate ctrl  Commented=on  a12=1 1/s  b2=1 1/m/s  k1=100 m  k2=20.5 m  N=5 m  kv=20  xv_specify=off  xv_priority=None  xv=0 m  xv_nominal_specify=off  xv_nominal_unit=m  xv_nominal_value=1  D1_specify=off  D1_priority=None  D1=0  D1_nominal_specify=off  D1_nominal_unit=1  D1_nominal_value=1  D2_specify=off  D2_priority=None  D2=0  D2_nominal_specify=off  D2_nominal_unit=1  D2_nominal_value=1
  PS-Simulink Converter : nesl_utility/PS-Simulink Converter  PhysicalDomain=network_engine_domain  SubClassName=ps_output  LeftPortType=input  RightPortType=output  PseudoPeriodic=off  Frequencies=[]  VectorFormat=1-D array  Unit=inherit  AffineConversion=off
  Scope : Scope  NumInputPorts=2
      settings: ActiveDisplayYMinimum=0.29414  ActiveDisplayYMaximum=1.07846  DataLoggingVariableName=ScopeData3
  Simulink-PS Converter3 : nesl_utility/Simulink-PS Converter  Commented=on  PhysicalDomain=network_engine_domain  SubClassName=ps_input  LeftPortType=input  RightPortType=output  PseudoPeriodic=off  Frequencies=[]  NoiseDistribution=none  NoiseParameters=[]  Unit=1  AffineConversion=off  FilteringAndDerivatives=provide  SimscapeFilterOrder=1  InputFilterTimeConstant=0.001  UdotUserProvided=0
  hose3 : Subsystem
  servo motor LD : Subsystem
  vd : PMIOPort  Side=Right
  pS : PMIOPort  Port=2  Side=Left
  pT : PMIOPort  Port=3  Side=Left
  wires:
  vd_ref/1 -> Simulink-PS Converter3/1, Scope/1, servo motor LD/1(displacement reference pu)
  PS-Simulink Converter/1 -> Scope/2
  connections:
  vd/RConn1 -- PS-Simulink Converter/LConn1 -- servo motor LD/RConn1
  hose3/RConn2 -- servo motor LD/LConn2
  hose3/RConn1 -- servo motor LD/LConn1
  pT/RConn1 -- hose3/LConn2
  pS/RConn1 -- hose3/LConn1
  Simulink-PS Converter3/RConn1 -- Linear swashplate ctrl2/LConn1

== system hdv_hydroelectropowertrain_model/PR776_powertrain/Hydrostatic_powertrain/driveine_LD2/vd_ctrl_pump_LD ==
  vd_ref : Inport
  Linear swashplate ctrl2 : linear_swashplate_ctrl_lib/Linear swashplate ctrl  Commented=on  a12=1 1/s  b2=1 1/m/s  k1=100 m  k2=20.5 m  N=5 m  kv=20  xv_specify=off  xv_priority=None  xv=0 m  xv_nominal_specify=off  xv_nominal_unit=m  xv_nominal_value=1  D1_specify=off  D1_priority=None  D1=0  D1_nominal_specify=off  D1_nominal_unit=1  D1_nominal_value=1  D2_specify=off  D2_priority=None  D2=0  D2_nominal_specify=off  D2_nominal_unit=1  D2_nominal_value=1
      settings: InternalSimscapePortConfiguration="{\"Bottom\":[],\"Left\":[{\"id\":\"D_ref\",\"label\":\"Dref\",\"type\":\"input\"}],\"Right\":[{\"id\":\"Dout\",\"label\":\"Dout\",\"type\":\"output\"}],\"Top\":[]}"
  Simulink-PS Converter3 : nesl_utility/Simulink-PS Converter  Commented=on  PhysicalDomain=network_engine_domain  SubClassName=ps_input  LeftPortType=input  RightPortType=output  PseudoPeriodic=off  Frequencies=[]  NoiseDistribution=none  NoiseParameters=[]  Unit=1  AffineConversion=off  FilteringAndDerivatives=provide  SimscapeFilterOrder=1  InputFilterTimeConstant=0.001  UdotUserProvided=0
  hose3 : Subsystem
  servo pump RD : Subsystem
  vd : PMIOPort  Side=Right
  pS : PMIOPort  Port=2  Side=Left
  pT : PMIOPort  Port=3  Side=Left
  wires:
  vd_ref/1 -> servo pump RD/1(displacement reference pu), Simulink-PS Converter3/1
  connections:
  servo pump RD/RConn1 -- vd/RConn1
  Simulink-PS Converter3/RConn1 -- Linear swashplate ctrl2/LConn1
  servo pump RD/LConn2 -- hose3/RConn2
  servo pump RD/LConn1 -- hose3/RConn1
  pS/RConn1 -- hose3/LConn1
  pT/RConn1 -- hose3/LConn2

== system hdv_hydroelectropowertrain_model/PR776_powertrain/Hydrostatic_powertrain/driveine_RD1/pressure_charge_system_RD ==
  Hydraulic Flow Rate Sensor : fl_lib/Hydraulic/Hydraulic Sensors/Hydraulic Flow Rate Sensor
  Hydraulic Flow Rate Sensor1 : fl_lib/Hydraulic/Hydraulic Sensors/Hydraulic Flow Rate Sensor
  Hydraulic Pressure Sensor{1..4} (4 alike) : fl_lib/Hydraulic/Hydraulic Sensors/Hydraulic Pressure Sensor
  Hydraulic Reference1 : fl_lib/Hydraulic/Hydraulic Elements/Hydraulic Reference
  Hydraulic Reference2 : fl_lib/Hydraulic/Hydraulic Elements/Hydraulic Reference
  Hydraulic Reference3 : fl_lib/Hydraulic/Hydraulic Elements/Hydraulic Reference
  Mux : Mux  Inputs=2
  PS-Simulink Converter : nesl_utility/PS-Simulink Converter  PhysicalDomain=network_engine_domain  SubClassName=ps_output  LeftPortType=input  RightPortType=output  PseudoPeriodic=off  Frequencies=[]  VectorFormat=1-D array  Unit=l/min  AffineConversion=on
  PS-Simulink Converter{1..3,5} (4 alike) : nesl_utility/PS-Simulink Converter  PhysicalDomain=network_engine_domain  SubClassName=ps_output  LeftPortType=input  RightPortType=output  PseudoPeriodic=off  Frequencies=[]  VectorFormat=1-D array  Unit=bar  AffineConversion=on
  PS-Simulink Converter4 : nesl_utility/PS-Simulink Converter  PhysicalDomain=network_engine_domain  SubClassName=ps_output  LeftPortType=input  RightPortType=output  PseudoPeriodic=off  Frequencies=[]  VectorFormat=1-D array  Unit=l/min  AffineConversion=on
  Scope1 : Scope  NumInputPorts=2
      settings: SampleTime=tsample  ActiveDisplayYMinimum=-11.94319  ActiveDisplayYMaximum=105.50779  DataLoggingVariableName=ScopeData2
  Scope2 : Scope  NumInputPorts=2
      settings: SampleTime=tsample  ActiveDisplayYMinimum=-1.41365  ActiveDisplayYMaximum=12.72285  DataLoggingVariableName=ScopeData2
  Subsystem : Subsystem
  hydro_check_valve1 : Subsystem
      settings: PortSchema="{\"entries\":[{\"content\":{\"sides\":[{\"content\":{\"connectorIds\":[]},\"type\":\"ConnectorPlacement.EquallySpacedRectSide\",\"uuid\":\"a69fbb91-2279-4dfd-af6f-16497d5f1538\"},{\"content\":{\"connectorIds\":[],\"side\":\"RIGHT\"},\"type\":\"ConnectorPlacement.EquallySpacedRectSide\",\"uuid\":\"52e95d44-b7af-4ccc-8556-a2abd2e724e0\"},{\"content\":{\"connectorIds\":[\"LConn1\"],\"side\":\"TOP\"},\"type\":\"ConnectorPlacement.EquallySpacedRectSide\",\"uuid\":\"2d8c071e-4cd0-4b83-8d45-c175cb858754\"},{\"content\":{\"connectorIds\":[\"RConn1\"],\"side\":\"BOTTOM\"},\"type\":\"ConnectorPlacement.EquallySpacedRectSide\",\"uuid\":\"1baec9dc-757c-4f21-904a-6fc08de72ce1\"}]},\"type\":\"ConnectorPlacement.EquallySpacedConnector\",\"uuid\":\"76990e53-6cb0-4bfe-8c9e-427c41b785f2\"}],\"packageUris\":[\"http://schema.mathworks.com/mf0/Connector/19700101\"],\"version\":\"1.0\"}"
  hydro_check_valve2 : Subsystem
      settings: PortSchema="{\"entries\":[{\"content\":{\"sides\":[{\"content\":{\"connectorIds\":[]},\"type\":\"ConnectorPlacement.EquallySpacedRectSide\",\"uuid\":\"a69fbb91-2279-4dfd-af6f-16497d5f1538\"},{\"content\":{\"connectorIds\":[],\"side\":\"RIGHT\"},\"type\":\"ConnectorPlacement.EquallySpacedRectSide\",\"uuid\":\"52e95d44-b7af-4ccc-8556-a2abd2e724e0\"},{\"content\":{\"connectorIds\":[\"LConn1\"],\"side\":\"TOP\"},\"type\":\"ConnectorPlacement.EquallySpacedRectSide\",\"uuid\":\"2d8c071e-4cd0-4b83-8d45-c175cb858754\"},{\"content\":{\"connectorIds\":[\"RConn1\"],\"side\":\"BOTTOM\"},\"type\":\"ConnectorPlacement.EquallySpacedRectSide\",\"uuid\":\"1baec9dc-757c-4f21-904a-6fc08de72ce1\"}]},\"type\":\"ConnectorPlacement.EquallySpacedConnector\",\"uuid\":\"76990e53-6cb0-4bfe-8c9e-427c41b785f2\"}],\"packageUris\":[\"http://schema.mathworks.com/mf0/Connector/19700101\"],\"version\":\"1.0\"}"
  inverse shuttle valve : inverse_shuttle_valve_lib/inverse shuttle valve  pnom=32 bar  dp_crack=0 bar  dp_reg=0 bar  x_rv_max=2 mm  a0=(2*pi*10)^2 1/s^2  a1=2*2*pi*10 1/s  leak=5e-12 m^3/s/Pa  qA_specify=off  qA_priority=None  qA=0 m^3/s  qA_nominal_specify=off  qA_nominal_unit=m^3/s  qA_nominal_value=1  qB_specify=off  qB_priority=None  qB=0 m^3/s  qB_nominal_specify=off  qB_nominal_unit=m^3/s  qB_nominal_value=1  qP_specify=off  qP_priority=None  qP=0 m^3/s  qP_nominal_specify=off  qP_nominal_unit=m^3/s  qP_nominal_value=1  dp_specify=off  dp_priority=None  dp=0 Pa  dp_nominal_specify=off  dp_nominal_unit=Pa  dp_nominal_value=1  dpAP_specify=off  dpAP_priority=None  dpAP=0 Pa  dpAP_nominal_specify=off  dpAP_nominal_unit=Pa  dpAP_nominal_value=1  dpBP_specify=off  dpBP_priority=None  dpBP=0 Pa  dpBP_nominal_specify=off  dpBP_nominal_unit=Pa  dpBP_nominal_value=1  x_rv_AP_specify=off  x_rv_AP_priority=None  x_rv_AP=0 m  x_rv_AP_nominal_specify=off  x_rv_AP_nominal_unit=m  x_rv_AP_nominal_value=1  x_rv_BP_specify=off  x_rv_BP_priority=None  x_rv_BP=0 m  x_rv_BP_nominal_specify=off  x_rv_BP_nominal_unit=m  x_rv_BP_nominal_value=1  x_rv_AP_flt_specify=off  x_rv_AP_flt_priority=None  x_rv_AP_flt=0 m  x_rv_AP_flt_nominal_specify=off  x_rv_AP_flt_nominal_unit=m  x_rv_AP_flt_nominal_value=1  x_rv_BP_flt_specify=off  x_rv_BP_flt_priority=None  x_rv_BP_flt=0 m  x_rv_BP_flt_nominal_specify=off  x_rv_BP_flt_nominal_unit=m  x_rv_BP_flt_nominal_value=1
  qt_ishuttle/dp : Scope  NumInputPorts=2
      settings: SampleTime=tsample  ActiveDisplayYMinimum=-2.35304  ActiveDisplayYMaximum=21.17734
  A : PMIOPort  Side=Left
  B : PMIOPort  Port=2  Side=Right
  D : PMIOPort  Port=3  Side=Right
  wires:
  PS-Simulink Converter2/1 -> Mux/2  "pA"
  PS-Simulink Converter1/1 -> Mux/1  "pB"
  Mux/1 -> Scope1/1
  PS-Simulink Converter/1 -> Scope1/2, Scope2/1  "qcharge"
  PS-Simulink Converter3/1 -> Scope2/2  "pCharge"
  PS-Simulink Converter4/1 -> qt_ishuttle/dp/1  "qt_ishuttle"
  PS-Simulink Converter5/1 -> qt_ishuttle/dp/2  "dp"
  connections:
  hydro_check_valve2/LConn1 -- Hydraulic Flow Rate Sensor/RConn2 -- hydro_check_valve1/LConn1
  A/RConn1 -- Hydraulic Pressure Sensor4/LConn1 -- inverse shuttle valve/LConn1 -- hydro_check_valve1/RConn1 -- Hydraulic Pressure Sensor2/LConn1
  B/RConn1 -- Hydraulic Pressure Sensor4/RConn1 -- inverse shuttle valve/LConn2 -- hydro_check_valve2/RConn1 -- Hydraulic Pressure Sensor1/LConn1
  Hydraulic Pressure Sensor2/RConn1 -- Hydraulic Reference1/LConn1 -- Hydraulic Pressure Sensor1/RConn1
  Hydraulic Pressure Sensor1/RConn2 -- PS-Simulink Converter1/LConn1
  Hydraulic Pressure Sensor2/RConn2 -- PS-Simulink Converter2/LConn1
  Hydraulic Flow Rate Sensor/RConn1 -- PS-Simulink Converter/LConn1
  Hydraulic Pressure Sensor3/LConn1 -- Subsystem/RConn1 -- Hydraulic Flow Rate Sensor/LConn1
  Subsystem/LConn1 -- D/RConn1
  Hydraulic Pressure Sensor3/RConn2 -- PS-Simulink Converter3/LConn1
  Hydraulic Reference2/LConn1 -- Hydraulic Pressure Sensor3/RConn1
  Hydraulic Flow Rate Sensor1/RConn2 -- Hydraulic Reference3/LConn1
  Hydraulic Flow Rate Sensor1/RConn1 -- PS-Simulink Converter4/LConn1
  PS-Simulink Converter5/LConn1 -- Hydraulic Pressure Sensor4/RConn2
  inverse shuttle valve/RConn1 -- Hydraulic Flow Rate Sensor1/LConn1

== system hdv_hydroelectropowertrain_model/PR776_powertrain/Hydrostatic_powertrain/driveine_RD1/vd_ctrl_motor_RD ==
  vd_ref : Inport
  Linear swashplate ctrl2 : linear_swashplate_ctrl_lib/Linear swashplate ctrl  Commented=on  a12=1 1/s  b2=1 1/m/s  k1=100 m  k2=20.5 m  N=5 m  kv=20  xv_specify=off  xv_priority=None  xv=0 m  xv_nominal_specify=off  xv_nominal_unit=m  xv_nominal_value=1  D1_specify=off  D1_priority=None  D1=0  D1_nominal_specify=off  D1_nominal_unit=1  D1_nominal_value=1  D2_specify=off  D2_priority=None  D2=0  D2_nominal_specify=off  D2_nominal_unit=1  D2_nominal_value=1
  PS-Simulink Converter : nesl_utility/PS-Simulink Converter  PhysicalDomain=network_engine_domain  SubClassName=ps_output  LeftPortType=input  RightPortType=output  PseudoPeriodic=off  Frequencies=[]  VectorFormat=1-D array  Unit=inherit  AffineConversion=off
  Scope : Scope  NumInputPorts=2
      settings: ActiveDisplayYMinimum=0.46161  ActiveDisplayYMaximum=1.05982  DataLoggingVariableName=ScopeData2
  Simulink-PS Converter3 : nesl_utility/Simulink-PS Converter  Commented=on  PhysicalDomain=network_engine_domain  SubClassName=ps_input  LeftPortType=input  RightPortType=output  PseudoPeriodic=off  Frequencies=[]  NoiseDistribution=none  NoiseParameters=[]  Unit=1  AffineConversion=off  FilteringAndDerivatives=provide  SimscapeFilterOrder=1  InputFilterTimeConstant=0.001  UdotUserProvided=0
  hose3 : Subsystem
  servo motor LD : Subsystem
  vd : PMIOPort  Side=Right
  pS : PMIOPort  Port=2  Side=Left
  pT : PMIOPort  Port=3  Side=Left
  wires:
  vd_ref/1 -> Scope/1, Simulink-PS Converter3/1, servo motor LD/1(displacement reference pu)
  PS-Simulink Converter/1 -> Scope/2
  connections:
  hose3/RConn2 -- servo motor LD/LConn2
  hose3/RConn1 -- servo motor LD/LConn1
  pS/RConn1 -- hose3/LConn1
  pT/RConn1 -- hose3/LConn2
  Simulink-PS Converter3/RConn1 -- Linear swashplate ctrl2/LConn1
  servo motor LD/RConn1 -- PS-Simulink Converter/LConn1 -- vd/RConn1

== system hdv_hydroelectropowertrain_model/PR776_powertrain/Hydrostatic_powertrain/driveine_RD1/vd_ctrl_pump_RD ==
  vd_ref : Inport
  Linear swashplate ctrl2 : linear_swashplate_ctrl_lib/Linear swashplate ctrl  Commented=on  a12=1 1/s  b2=1 1/m/s  k1=100 m  k2=20.5 m  N=5 m  kv=20  xv_specify=off  xv_priority=None  xv=0 m  xv_nominal_specify=off  xv_nominal_unit=m  xv_nominal_value=1  D1_specify=off  D1_priority=None  D1=0  D1_nominal_specify=off  D1_nominal_unit=1  D1_nominal_value=1  D2_specify=off  D2_priority=None  D2=0  D2_nominal_specify=off  D2_nominal_unit=1  D2_nominal_value=1
  Simulink-PS Converter3 : nesl_utility/Simulink-PS Converter  Commented=on  PhysicalDomain=network_engine_domain  SubClassName=ps_input  LeftPortType=input  RightPortType=output  PseudoPeriodic=off  Frequencies=[]  NoiseDistribution=none  NoiseParameters=[]  Unit=1  AffineConversion=off  FilteringAndDerivatives=provide  SimscapeFilterOrder=1  InputFilterTimeConstant=0.001  UdotUserProvided=0
  hose3 : Subsystem
  servo pump RD : Subsystem
  vd : PMIOPort  Side=Right
  pS : PMIOPort  Port=2  Side=Left
  pT : PMIOPort  Port=3  Side=Left
  wires:
  vd_ref/1 -> servo pump RD/1(displacement reference pu), Simulink-PS Converter3/1
  connections:
  servo pump RD/LConn2 -- hose3/RConn2
  servo pump RD/LConn1 -- hose3/RConn1
  pS/RConn1 -- hose3/LConn1
  pT/RConn1 -- hose3/LConn2
  Simulink-PS Converter3/RConn1 -- Linear swashplate ctrl2/LConn1
  servo pump RD/RConn1 -- vd/RConn1
